simulink model "quartercarmodel"  (R2025a)
settings: Solver=VariableStepAuto  StartTime=0.0  StopTime=10.0  RelTol=1e-3
undefined symbols (not defined in the file): c1, k1, k2, mc, ms
settings Model: Creator=krishDragneel  LastModifiedBy=krishDragneel

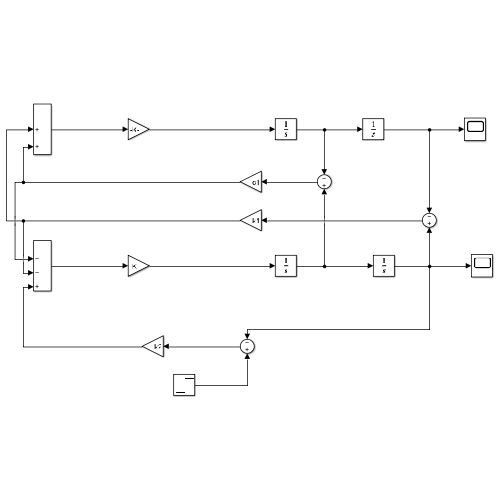
[thumbnail: Simulink's stored preview of the top-level diagram]
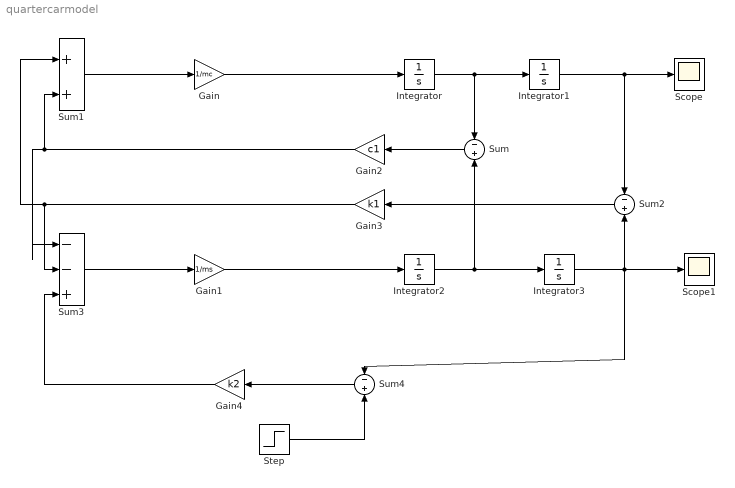
== system quartercarmodel ==
  Gain : Gain  Gain=1/mc
  Gain1 : Gain  Gain=1/ms
  Gain2 : Gain  Gain=c1
  Gain3 : Gain  Gain=k1
  Gain4 : Gain  Gain=k2
  Integrator{,1..3} (4 alike) : Integrator
  Scope : Scope
      settings: ActiveDisplayYMinimum=-5.1852029753195223  ActiveDisplayYMaximum=46.666826777875713
  Scope1 : Scope
  Step : Step  After=30  SampleTime=0
  Sum : Sum  Inputs=-+
  Sum1 : Sum  Inputs=|++
  Sum2 : Sum  Inputs=-+
  Sum3 : Sum  Inputs=|--+
  Sum4 : Sum  Inputs=-+
  wires:
  Gain/1 -> Integrator/1
  Integrator/1 -> Integrator1/1, Sum/1
  Integrator1/1 -> Sum2/1, Scope/1
  Gain1/1 -> Integrator2/1
  Integrator2/1 -> Integrator3/1, Sum/2
  Integrator3/1 -> Sum4/1, Scope1/1, Sum2/2
  Sum/1 -> Gain2/1
  Sum2/1 -> Gain3/1
  Gain2/1 -> Sum3/1, Sum1/2
  Gain3/1 -> Sum3/2, Sum1/1
  Sum1/1 -> Gain/1
  Sum3/1 -> Gain1/1
  Step/1 -> Sum4/2
  Sum4/1 -> Gain4/1
  Gain4/1 -> Sum3/3
